simulink model "BouncingBallModel"  (R2021b)
settings: Solver=VariableStepAuto  StartTime=0.0  StopTime=10.0  RelTol=1e-3
libraries: vrlib x2
settings Model: Creator=omkar  LastModifiedBy=omkar

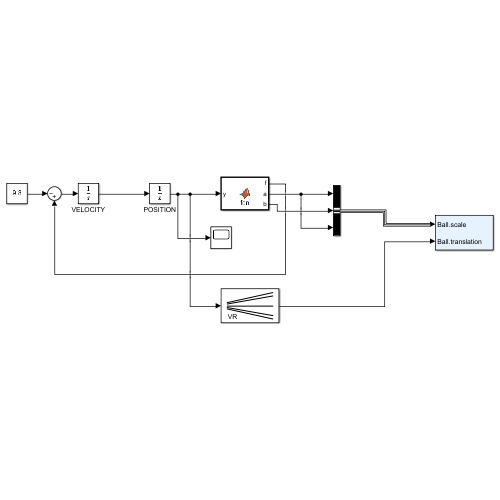
[thumbnail: Simulink's stored preview of the top-level diagram]
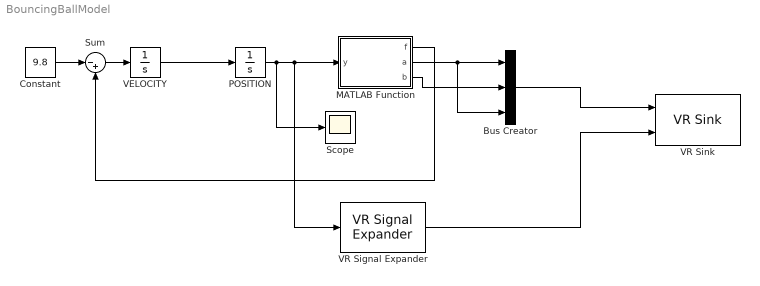
== system BouncingBallModel ==
  Bus Creator : BusCreator  Inputs=3
  Constant : Constant  Value=9.8
  MATLAB Function : MATLAB Function  TreatAsAtomicUnit=on
  POSITION : Integrator  InitialCondition=20
  Scope : Scope
  Sum : Sum  Inputs=|-+
  VELOCITY : Integrator
  VR Signal Expander : vrlib/VR Signal Expander  outwidth=3  outidx=[2]
  VR Sink : vrlib/VR Sink  InstantiateOnLoad=on  SampleTime=0.01  ViewEnable=on  RemoteChange=off  RemoteView=off  FieldsWritten=Ball.scale.3.1.1.double#Ball.translation.3.1.1.double  WorldFileName=bouncing_ball.x3d  AutoView=off  VideoDimensions=[]  AllowVariableSize=off  FigureProperties="{'Position', 'Name', 'Viewpoint', 'CameraBound', 'CameraDirection', 'CameraPosition', 'CameraUpVector', 'ZoomFactor', 'Antialiasing', 'Headlight', 'Lighting', 'NavPanel', 'Sound', 'StatusBar', 'Stereo3D', 'Stereo3DCameraOffset', 'Stereo3DHIT', 'ToolBar', 'Textures', 'Transparency', 'Triad', 'Wireframe', 'NavZones', 'NavMode', 'NavSpeed', 'CaptureFileFormat', 'CaptureFileName', 'Record2DCompressMethod', 'Record2DCompressQuality', 'Record2D', 'Record2DFileName', 'Record2DFPS'; [8.6820000000000005e+02   2.3979999999999995e+02   5.7600000000000000e+02   3.5000000000000000e+02], '', '_untitled_1', 'on', [0.0000000000000000e+00   0.0000000000000000e+00  -1.0000000000000000e+00], [0.0000000000000000e+00   0.0000000000000000e+00   6.7000000000000000e+01], [0.0000000000000000e+00   1.0000000000000000e+00   0.0000000000000000e+00], [1.0000000000000000e+00], 'on', 'on', 'on', 'halfbar', 'on', 'on', 'off', [1.0000000149011612e-01], [0.0000000000000000e+00], 'on', 'on', 'on', 'none', 'off', 'off', 'fly', 'normal', 'tif', '%f_anim_%n.tif', 'auto', [7.5000000000000000e+01], 'off', '%f_anim_%n.avi', 'auto'}"
  wires:
  Constant/1 -> Sum/1
  VELOCITY/1 -> POSITION/1
  POSITION/1 -> Scope/1, VR Signal Expander/1, MATLAB Function/1(y)
  MATLAB Function/1(f) -> Sum/2
  Sum/1 -> VELOCITY/1
  MATLAB Function/2(a) -> Bus Creator/3, Bus Creator/1
  MATLAB Function/3(b) -> Bus Creator/2
  VR Signal Expander/1 -> VR Sink/2
  Bus Creator/1 -> VR Sink/1

== matlab function BouncingBallModel/MATLAB Function ==
  data: y input; f output; a output; b output
function [f, a, b] = fcn(y)

if y<1e-4
    y=1e-4;
end

if y<1.5
    f=500*(1.5-y);
    a=sqrt(1.5^3/y);
    b=y;
else
    f=0;
    a=1.5;
    b=1.5;
end
